simulink model "Model_RB_APF_WF_VO_withFairRules"  (R2024b)
settings: Solver=FixedStepAuto  StartTime=0.0  StopTime=150  FixedStep=UAVSampleTime  RelTol=1e-3
undefined symbols (not defined in the file): DroneMass, Gravity, Horizontal_Limits, Horizontal_Res, kD_pos, kD_vel, kI_pos, kI_vel, kP_pos, kP_vel, Lidar, MaxRange, N_filter, TopSpeed, UAV, Vertical_Limits, Vertical_Res, Waypoints
libraries: slpidlib x6, uavsimlib x4, robotcorelib x1, uavalgslib x1
(part 1 of 2)
settings Model: NumberOfSteps=100  PacingRate=10  Creator=The MathWorks, Inc.  LastModifiedBy=phill
settings SolverCC: AlgebraicLoopSolver=TrustRegion
settings DebuggingCC: ParameterPrecisionLossMsg=none  UnconnectedInputMsg=warning  UnconnectedOutputMsg=warning  UnconnectedLineMsg=warning
settings ModelReferenceCC: EnableRefExpFcnMdlSchedulingChecks=on
settings RTWCC: GPUComputeCapability=3.5  DLArmComputeVersion=19.05

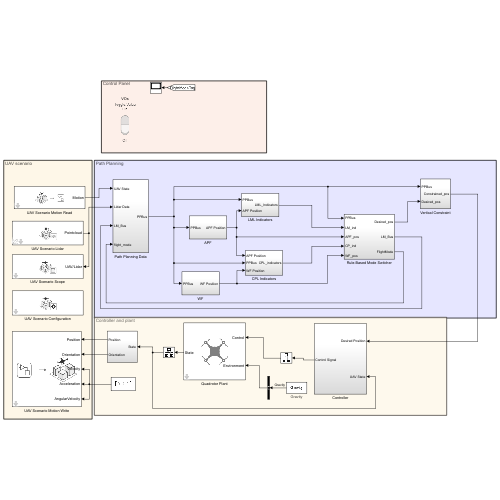
[thumbnail: Simulink's stored preview of the top-level diagram]
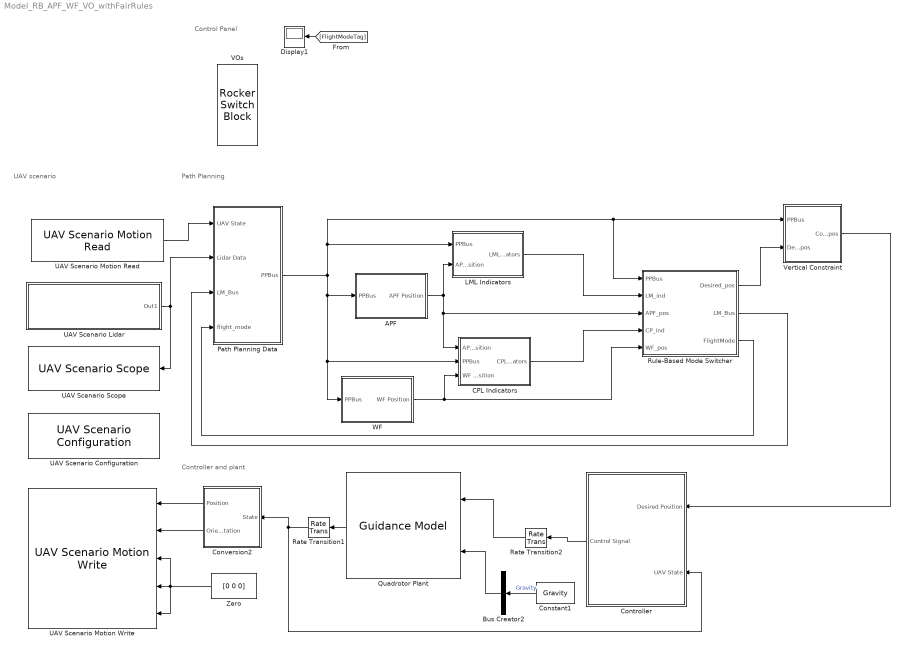
== system Model_RB_APF_WF_VO_withFairRules ==
  note: Path Planning
  note: UAV scenario
  note: Controller and plant
  note: Control Panel
  APF : Subsystem
  Bus Creator2 : BusCreator  Inputs=1  OutDataTypeStr=Bus: uavGuidanceEnvironmentBus  NonVirtualBus=on
  CPL Indicators : Subsystem
  Constant1 : Constant  Value=Gravity  OutDataTypeStr=single
      settings: AttributesFormatString=%<Value>
  Controller : Subsystem
  Conversion2 : Subsystem
  Display1 : Display
  LML Indicators : Subsystem
  Path Planning Data : Subsystem
  Quadrotor Plant : uavalgslib/Guidance Model  ModelType=MultirotorGuidance  SpecifiedDataType=single  SimulateUsing=Code generation  InitialWorldPositionMultirotor=InitialPosition'  InitialWorldVelocityMultirotor=[0; 0; 0]  InitialEulerZYXMultirotor=|  InitialBodyAngularRateRPYMultirotor=[0; 0; 0]  InitialThrustMultirotor=0  InitialNorthFixedWing=0  InitialEastFixedWing=0  InitialHeightFixedWing=0  InitialAirSpeedFixedWing=0  InitialHeadingAngleFixedWing=0  InitialFlightPathAngleFixedWing=0  InitialRollAngleFixedWing=0  InitialRollAngleRateFixedWing=0  PDRollMultirotor=[100,10]  PDPitchMultirotor=[100,10]  PYawRateMultirotor=50  PThrustMultirotor=100  MassMultirotor=0.1  PHeightFixedWing=3.9  PHeadingAngleFixedWing=3.9  PFlightPathAngleFixedWing=39  PDRollFixedWing=[3402.97, 116.67]  PAirSpeedFixedWing=1  FlightPathAngleLimitsFixedWing=[-pi/2, pi/2]  StateBusName='uavGuidanceStateBus'  ControlBusName='uavGuidanceControlBus'  EnvironmentBusName='uavGuidanceEnvironmentBus'  DataType=single
      | [ 0
      | ;0;0]
  Rate Transition1 : RateTransition  OutPortSampleTime=UAVSampleTime
  Rate Transition2 : RateTransition  OutPortSampleTime=UAVSampleTime
  Rule-Based Mode Switcher : Subsystem
  UAV Scenario Configuration : uavsimlib/UAV Scenario Configuration  Priority=-1  UAVScenarioObject=MyScenario  SampleTime=0.1  UpdateParam=true  SensorMotionBusName='SensorMotionBus'  PlatformMotionBusName='PlatformMotionBus'  ScenarioMotionBusName='ScenarioMotionBus'  ScenarioMotionSignalName='ScenarioMotions'
  UAV Scenario Lidar : Subsystem  Priority=1  AncestorBlock=uavsimlib/UAV Scenario Lidar  mask(UAV Scenario Lidar){SensorName=UAV/Lidar, MaxRange=MaxRange, RangeAccuracy=0.02, AzimuthLimits=Horizontal_Limits, AzimuthResolution=Horizontal_Res, ElevationLimits=Vertical_Limits, ElevationResolution=Vertical_Res, HasNoise=off, HasOrganizedOutput=on, SampleTime=0.1}
      mask prompts: SensorName "uav:robotsluav:uavscenariolidar:SensorName"; MaxRange "uav:robotsluav:uavscenariolidar:MaxRange"; RangeAccuracy "uav:robotsluav:uavscenariolidar:RangeAccuracy"; AzimuthLimits "uav:robotsluav:uavscenariolidar:AzimuthLimits"; AzimuthResolution "uav:robotsluav:uavscenariolidar:AzimuthResolution"; ElevationLimits "uav:robotsluav:uavscenariolidar:ElevationLimits"; ElevationResolution "uav:robotsluav:uavscenariolidar:ElevationResolution"; HasNoise "uav:robotsluav:uavscenariolidar:HasNoise"; HasOrganizedOutput "uav:robotsluav:uavscenariolidar:HasOrganizedOutput"; SampleTime "uav:robotsluav:uavscenariolidar:SampleTime"
      mask help: uav:robotsluav:uavscenariolidar:Description
      mask init:
      | % Need to set sample time to a valid value before initializing with
      | % additional set_param calls
      | set_param([gcb, '/MotionData'], 'SampleTime', '-1');
      | dataSampleTime = uav.sluav.internal.scenario.mask.ScenarioLidarSensor.initialize(gcb);
      | set_param([gcb, '/MotionData'], 'SampleTime', 'dataSampleTime');
      mask Help: eval('helpview("uav","uavScenarioLidar")');
      mask TypeOptions SensorName: LidarSensor/SensorName
      mask TypeOptions MaxRange: LidarSensor/MaxRange
      mask TypeOptions RangeAccuracy: LidarSensor/RangeAccuracy
      mask TypeOptions AzimuthLimits: LidarSensor/AzimuthLimits
      mask TypeOptions AzimuthResolution: LidarSensor/AzimuthResolution
      mask TypeOptions ElevationLimits: LidarSensor/ElevationLimits
      mask TypeOptions ElevationResolution: LidarSensor/ElevationResolution
      mask TypeOptions HasNoise: LidarSensor/HasNoise
      mask TypeOptions HasOrganizedOutput: LidarSensor/HasOrganizedOutput
      mask TypeOptions SampleTime: LidarSensor/SampleTime
      mask DialogControl SensorName Prompt: Sensor name:
      mask DialogControl SelectBtn Prompt: uav:robotsluav:uavscenarioconfig:SelectBtnPrompt
      mask DialogControl SelectBtn Callback: uav.sluav.internal.scenario.mask.ScenarioLidarSensor.selectBtnCallback(gcb);
      mask DialogControl MaxRange Prompt: Max range (m):
      mask DialogControl RangeAccuracy Prompt: Range accuracy (m):
      mask DialogControl AzimuthLimits Prompt: Azimuthal limits (deg):
      mask DialogControl AzimuthResolution Prompt: Azimuthal resolution (deg):
      mask DialogControl ElevationLimits Prompt: Elevation limits (deg):
      mask DialogControl ElevationResolution Prompt: Elevation resolution (deg):
      mask DialogControl HasNoise Prompt: Add noise to measurement.
      mask DialogControl HasOrganizedOutput Prompt: Output organized point cloud locations.
      mask DialogControl SampleTime Prompt: Sample Time:
      mask Display: port_label('output', 1, 'Pointcloud');
  UAV Scenario Motion Read : uavsimlib/UAV Scenario Motion Read  Priority=1  EntityName='UAV'  ReferenceFrame=ENU  OutputWind=off
  UAV Scenario Motion Write : uavsimlib/UAV Scenario Motion Write  Priority=0  PlatName='UAV'  ReferenceFrame=ENU
  UAV Scenario Scope : uavsimlib/UAV Scenario Scope  Priority=1  SensorNameTable={ 'UAV/Lidar', 'on' }  SampleTime=.1
  VOs : RockerSwitchBlock
      settings: Values={{'Off', 'On'}, [0 1]}
  Vertical Constraint : Subsystem
  WF : Subsystem
  Zero : Constant  Value=[0 0 0]  OutDataTypeStr=Inherit: Inherit via back propagation
  wires:
  Controller/1(Control Signal) -> Rate Transition2/1
  Rate Transition2/1 -> Quadrotor Plant/1
  Rate Transition1/1 -> Controller/2(UAV State), Conversion2/1(State)
  Quadrotor Plant/1 -> Rate Transition1/1
  Bus Creator2/1 -> Quadrotor Plant/2
  Constant1/1 -> Bus Creator2/1  "Gravity"
  UAV Scenario Motion Read/1 -> Path Planning Data/1(UAV State)
  UAV Scenario Lidar/1(Out1) -> UAV Scenario Scope/1, Path Planning Data/2(Lidar Data)
  Conversion2/1(Position) -> UAV Scenario Motion Write/1
  Conversion2/2(Orientation) -> UAV Scenario Motion Write/2
  Zero/1 -> UAV Scenario Motion Write/3, UAV Scenario Motion Write/4, UAV Scenario Motion Write/5
  APF/1(APF Position) -> Rule-Based Mode Switcher/3(APF_pos), CPL Indicators/1(APF Position), LML Indicators/2(APF Position)
  WF/1(WF Position) -> Rule-Based Mode Switcher/5(WF_pos), CPL Indicators/3(WF Position)
  Vertical Constraint/1(Constrained_pos) -> Controller/1(Desired Position)
  [FlightModeTag] -> Display1/1
  Path Planning Data/1(PPBus) -> LML Indicators/1(PPBus), Rule-Based Mode Switcher/1(PPBus), Vertical Constraint/1(PPBus), CPL Indicators/2(PPBus), WF/1(PPBus), APF/1(PPBus)
  CPL Indicators/1(CPL_indicators) -> Rule-Based Mode Switcher/4(CP_ind)
  Rule-Based Mode Switcher/1(Desired_pos) -> Vertical Constraint/2(Desired_pos)
  Rule-Based Mode Switcher/3(FlightMode) -> Path Planning Data/4(flight_mode)
  Rule-Based Mode Switcher/2(LM_Bus) -> Path Planning Data/3(LM_Bus)
  LML Indicators/1(LML_Indicators) -> Rule-Based Mode Switcher/2(LM_ind)

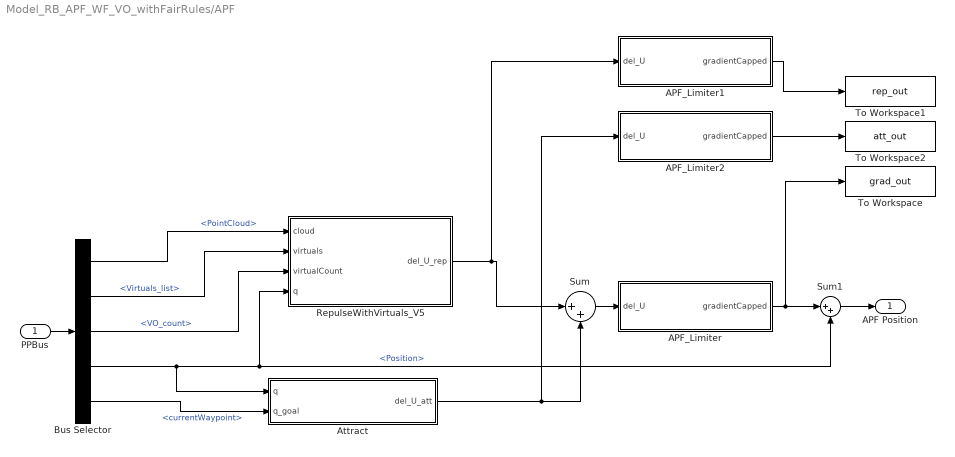
== system Model_RB_APF_WF_VO_withFairRules/APF ==
  PPBus : Inport
  APF_Limiter : MATLAB Function  TreatAsAtomicUnit=on
  APF_Limiter1 : MATLAB Function  TreatAsAtomicUnit=on
  APF_Limiter2 : MATLAB Function  TreatAsAtomicUnit=on
  Attract : MATLAB Function  TreatAsAtomicUnit=on
  Bus Selector : BusSelector  OutputSignals=PointCloud,VO_Bus.Virtuals_list,VO_Bus.VO_count,Position,currentWaypoint
  RepulseWithVirtuals_V5 : MATLAB Function  TreatAsAtomicUnit=on
  Sum : Sum  Inputs=|++
  Sum1 : Sum  Inputs=|++
  To Workspace : ToWorkspace  VariableName=grad_out  SampleTime=-1
      settings: Decimation=Plot_decimation_1s
  To Workspace1 : ToWorkspace  VariableName=rep_out  SampleTime=-1
      settings: Decimation=Plot_decimation_1s
  To Workspace2 : ToWorkspace  VariableName=att_out  SampleTime=-1
      settings: Decimation=Plot_decimation_1s
  APF Position : Outport
  wires:
  PPBus/1 -> Bus Selector/1
  Sum1/1 -> APF Position/1
  Sum/1 -> APF_Limiter/1(del_U)
  APF_Limiter/1(gradientCapped) -> Sum1/1, To Workspace/1
  Attract/1(del_U_att) -> APF_Limiter2/1(del_U), Sum/2
  RepulseWithVirtuals_V5/1(del_U_rep) -> APF_Limiter1/1(del_U), Sum/1
  Bus Selector/1 -> RepulseWithVirtuals_V5/1(cloud)  "<PointCloud>"
  Bus Selector/4 -> RepulseWithVirtuals_V5/4(q), Sum1/2, Attract/1(q)  "<Position>"
  Bus Selector/5 -> Attract/2(q_goal)  "<currentWaypoint>"
  APF_Limiter1/1(gradientCapped) -> To Workspace1/1
  APF_Limiter2/1(gradientCapped) -> To Workspace2/1
  Bus Selector/2 -> RepulseWithVirtuals_V5/2(virtuals)  "<Virtuals_list>"
  Bus Selector/3 -> RepulseWithVirtuals_V5/3(virtualCount)  "<VO_count>"

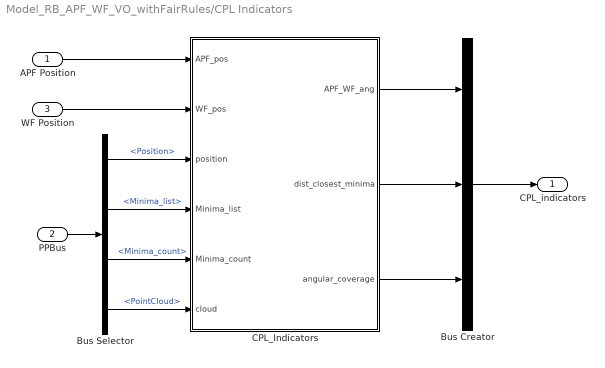
== system Model_RB_APF_WF_VO_withFairRules/CPL Indicators ==
  APF Position : Inport
  PPBus : Inport  Port=2
  WF Position : Inport  Port=3
  Bus Creator : BusCreator  Inputs=3
  Bus Selector : BusSelector  OutputSignals=Position,LM_Bus.Minima_list,LM_Bus.Minima_count,PointCloud
  CPL_Indicators : MATLAB Function  TreatAsAtomicUnit=on
  CPL_indicators : Outport
  wires:
  PPBus/1 -> Bus Selector/1
  Bus Selector/1 -> CPL_Indicators/3(position)  "<Position>"
  Bus Selector/3 -> CPL_Indicators/5(Minima_count)  "<Minima_count>"
  Bus Selector/2 -> CPL_Indicators/4(Minima_list)  "<Minima_list>"
  Bus Selector/4 -> CPL_Indicators/6(cloud)  "<PointCloud>"
  Bus Creator/1 -> CPL_indicators/1
  CPL_Indicators/2(dist_closest_minima) -> Bus Creator/2
  CPL_Indicators/3(angular_coverage) -> Bus Creator/3
  WF Position/1 -> CPL_Indicators/2(WF_pos)
  APF Position/1 -> CPL_Indicators/1(APF_pos)
  CPL_Indicators/1(APF_WF_ang) -> Bus Creator/1

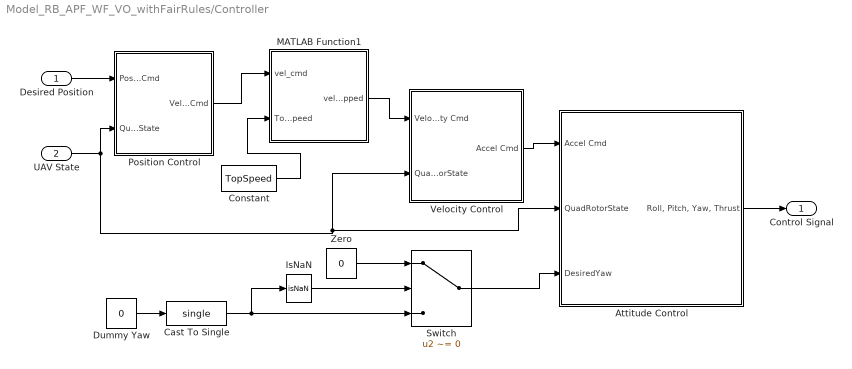
== system Model_RB_APF_WF_VO_withFairRules/Controller ==
  Desired Position : Inport
  UAV State : Inport  Port=2
  Attitude Control : Subsystem
  Cast To Single : DataTypeConversion  OutDataTypeStr=single  SaturateOnIntegerOverflow=off  RndMeth=Floor
  Constant : Constant  Value=TopSpeed
  Dummy Yaw : Constant  Value=0
  IsNaN : RelationalOperator  Operator=isNaN  OutDataTypeStr=boolean  RndMeth=Simplest  InputSameDT=off
  MATLAB Function1 : MATLAB Function  TreatAsAtomicUnit=on
  Position Control : Subsystem
  Switch : Switch  Criteria=u2 ~= 0  SaturateOnIntegerOverflow=off  InputSameDT=off
  Velocity Control : Subsystem
  Zero : Constant  Value=0  OutDataTypeStr=Inherit: Inherit via back propagation
  Control Signal : Outport
  wires:
  Desired Position/1 -> Position Control/1(PositionCmd)
  Velocity Control/1(Accel Cmd) -> Attitude Control/1(Accel Cmd)
  Attitude Control/1("Roll, Pitch, Yaw, Thrust") -> Control Signal/1
  UAV State/1 -> Position Control/2(QuadRotorState), Velocity Control/2(QuadRotorState), Attitude Control/2(QuadRotorState)
  Zero/1 -> Switch/1
  IsNaN/1 -> Switch/2
  Cast To Single/1 -> IsNaN/1, Switch/3
  Switch/1 -> Attitude Control/3(DesiredYaw)
  Dummy Yaw/1 -> Cast To Single/1
  Position Control/1(Velocity Cmd) -> MATLAB Function1/1(vel_cmd)
  MATLAB Function1/1(vel_capped) -> Velocity Control/1(Velocity Cmd)
  Constant/1 -> MATLAB Function1/2(TopSpeed)

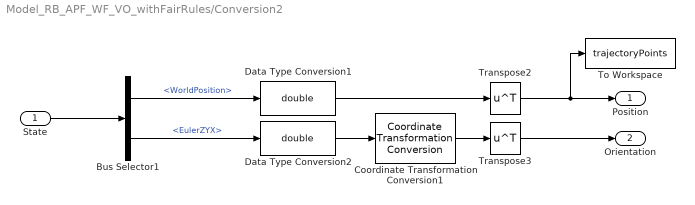
== system Model_RB_APF_WF_VO_withFairRules/Conversion2 ==
  State : Inport
  Bus Selector1 : BusSelector  OutputSignals=WorldPosition,EulerZYX
  Coordinate Transformation Conversion1 : robotcorelib/Coordinate Transformation Conversion  InputRepresentation=Euler Angles  InputEulerSequence=ZYX  ShowTrVecInputPort=on  OutputRepresentation=Quaternion  OutputEulerSequence=ZYX  ShowTrVecOutputPort=on  SimulateUsing=Code generation
  Data Type Conversion1 : DataTypeConversion  OutDataTypeStr=double  SaturateOnIntegerOverflow=off  RndMeth=Floor
  Data Type Conversion2 : DataTypeConversion  OutDataTypeStr=double  SaturateOnIntegerOverflow=off  RndMeth=Floor
  To Workspace : ToWorkspace  VariableName=trajectoryPoints  SampleTime=-1
  Transpose2 : Math  Operator=transpose
  Transpose3 : Math  Operator=transpose
  Position : Outport
  Orientation : Outport  Port=2
  wires:
  State/1 -> Bus Selector1/1
  Transpose2/1 -> To Workspace/1, Position/1
  Bus Selector1/1 -> Data Type Conversion1/1  "<WorldPosition>"
  Data Type Conversion2/1 -> Coordinate Transformation Conversion1/1
  Bus Selector1/2 -> Data Type Conversion2/1  "<EulerZYX>"
  Coordinate Transformation Conversion1/1 -> Transpose3/1
  Transpose3/1 -> Orientation/1
  Data Type Conversion1/1 -> Transpose2/1

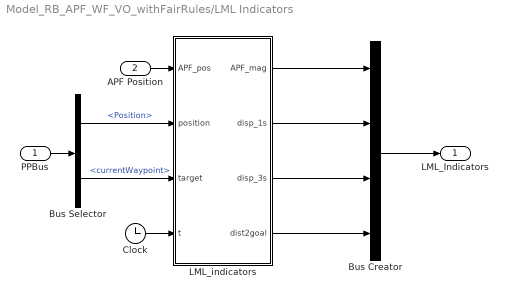
== system Model_RB_APF_WF_VO_withFairRules/LML Indicators ==
  PPBus : Inport
  APF Position : Inport  Port=2
  Bus Creator : BusCreator  Inputs=4
  Bus Selector : BusSelector  OutputSignals=Position,currentWaypoint
  Clock : Clock
  LML_indicators : MATLAB Function  TreatAsAtomicUnit=on
  LML_Indicators : Outport
  wires:
  PPBus/1 -> Bus Selector/1
  Bus Selector/1 -> LML_indicators/2(position)  "<Position>"
  Clock/1 -> LML_indicators/4(t)
  LML_indicators/3(disp_3s) -> Bus Creator/3
  LML_indicators/2(disp_1s) -> Bus Creator/2
  APF Position/1 -> LML_indicators/1(APF_pos)
  LML_indicators/1(APF_mag) -> Bus Creator/1
  Bus Creator/1 -> LML_Indicators/1
  Bus Selector/2 -> LML_indicators/3(target)  "<currentWaypoint>"
  LML_indicators/4(dist2goal) -> Bus Creator/4

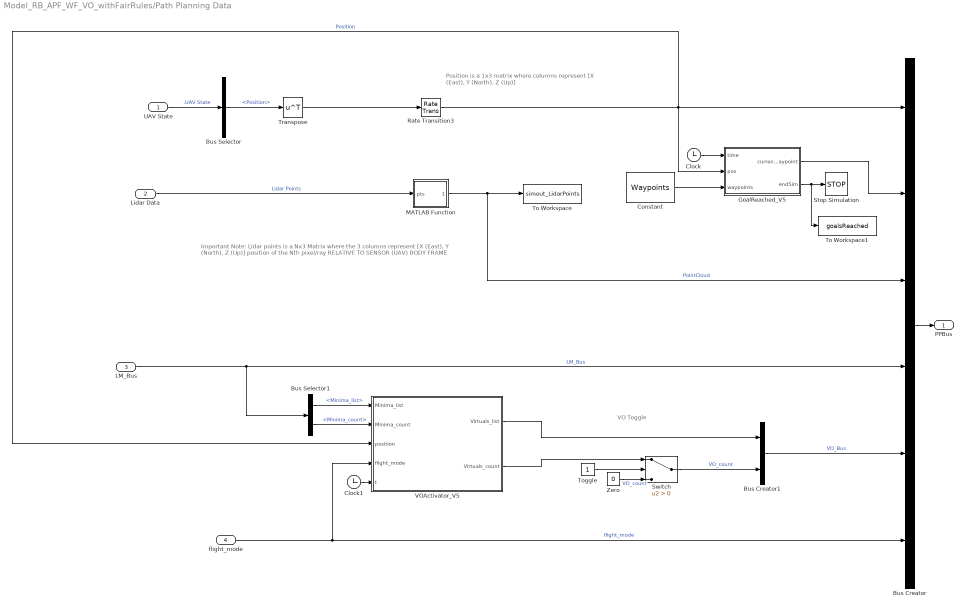
== system Model_RB_APF_WF_VO_withFairRules/Path Planning Data ==
  note: VO Toggle
  note: Position is a 1x3 matrix where columns represent [X (East), Y (North), Z (Up)]
  note: Important Note:
      | Lidar points is a Nx3 Matrix where the 3 columns represent [X (East), Y (North), Z (Up)] position of the Nth pixel/ray RELATIVE TO SENSOR (UAV) BODY FRAME
  UAV State : Inport
  Lidar Data : Inport  Port=2
  LM_Bus : Inport  Port=3
  flight_mode : Inport  Port=4
  Bus Creator : BusCreator  Inputs=6
  Bus Creator1 : BusCreator  Inputs=2
  Bus Selector : BusSelector  OutputSignals=Position
  Bus Selector1 : BusSelector  OutputSignals=Minima_list,Minima_count
  Clock : Clock
  Clock1 : Clock
  Constant : Constant  Value=Waypoints  VectorParams1D=off
  GoalReached_V5 : MATLAB Function  TreatAsAtomicUnit=on
  MATLAB Function : MATLAB Function  TreatAsAtomicUnit=on
  Rate Transition3 : RateTransition  OutPortSampleTime=.1
  Stop Simulation : Stop
  Switch : Switch  Criteria=u2 > Threshold  SaturateOnIntegerOverflow=off  InputSameDT=off
  To Workspace : ToWorkspace  VariableName=simout_LidarPoints  SampleTime=-1
  To Workspace1 : ToWorkspace  VariableName=goalsReached  SaveFormat=Timeseries  SampleTime=-1
  Toggle : Constant
  Transpose : Math  Operator=transpose
  VOActivator_V5 : MATLAB Function  TreatAsAtomicUnit=on
  Zero : Constant  Value=0
  PPBus : Outport
  wires:
  Bus Selector/1 -> Transpose/1  "<Position>"
  UAV State/1 -> Bus Selector/1  ".UAV State"
  Lidar Data/1 -> MATLAB Function/1(pts)  "Lidar Points"
  MATLAB Function/1(points) -> Bus Creator/3, To Workspace/1  "PointCloud"
  Rate Transition3/1 -> GoalReached_V5/2(pos), VOActivator_V5/3(position), Bus Creator/1  "Position"
  Transpose/1 -> Rate Transition3/1
  Bus Creator/1 -> PPBus/1
  Constant/1 -> GoalReached_V5/3(waypoints)
  Clock/1 -> GoalReached_V5/1(time)
  Toggle/1 -> Switch/2
  Switch/1 -> Bus Creator1/2  "VO_count"
  Zero/1 -> Switch/3  "VO_count"
  Bus Creator1/1 -> Bus Creator/5  "VO_Bus"
  LM_Bus/1 -> Bus Selector1/1, Bus Creator/4  "LM_Bus"
  VOActivator_V5/1(Virtuals_list) -> Bus Creator1/1
  VOActivator_V5/2(Virtuals_count) -> Switch/1
  flight_mode/1 -> VOActivator_V5/4(flight_mode), Bus Creator/6  "flight_mode"
  Bus Selector1/1 -> VOActivator_V5/1(Minima_list)  "<Minima_list>"
  Bus Selector1/2 -> VOActivator_V5/2(Minima_count)  "<Minima_count>"
  Clock1/1 -> VOActivator_V5/5(t)
  GoalReached_V5/1(currentWaypoint) -> Bus Creator/2
  GoalReached_V5/2(endSim) -> To Workspace1/1, Stop Simulation/1

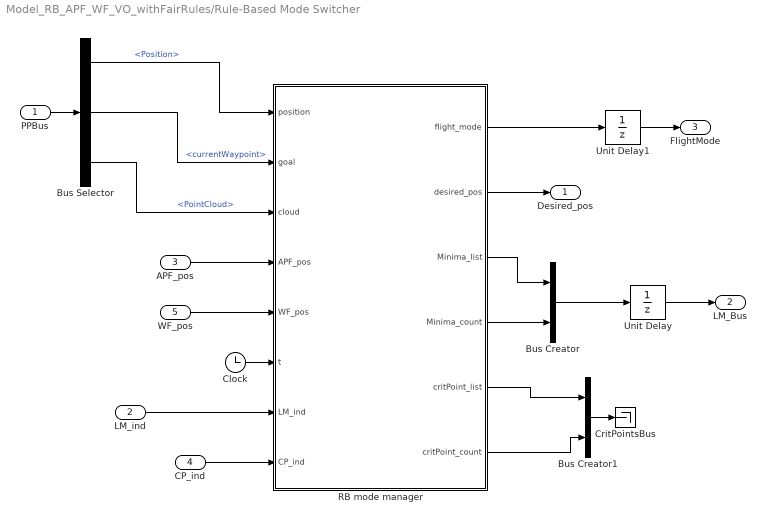
== system Model_RB_APF_WF_VO_withFairRules/Rule-Based Mode Switcher ==
  PPBus : Inport
  LM_ind : Inport  Port=2
  APF_pos : Inport  Port=3
  CP_ind : Inport  Port=4
  WF_pos : Inport  Port=5
  Bus Creator : BusCreator  Inputs=2
  Bus Creator1 : BusCreator  Inputs=2
  Bus Selector : BusSelector  OutputSignals=Position,currentWaypoint,PointCloud
  Clock : Clock
  CritPointsBus : Terminator
  RB mode manager : MATLAB Function  TreatAsAtomicUnit=on
  Unit Delay : UnitDelay  InitialCondition=1  SampleTime=-1  HasFrameUpgradeWarning=on
  Unit Delay1 : UnitDelay  InitialCondition=1  SampleTime=-1  HasFrameUpgradeWarning=on
  Desired_pos : Outport
  LM_Bus : Outport  Port=2
  FlightMode : Outport  Port=3
  wires:
  APF_pos/1 -> RB mode manager/4(APF_pos)
  WF_pos/1 -> RB mode manager/5(WF_pos)
  PPBus/1 -> Bus Selector/1
  Bus Selector/1 -> RB mode manager/1(position)  "<Position>"
  Bus Selector/2 -> RB mode manager/2(goal)  "<currentWaypoint>"
  Bus Selector/3 -> RB mode manager/3(cloud)  "<PointCloud>"
  RB mode manager/2(desired_pos) -> Desired_pos/1
  RB mode manager/3(Minima_list) -> Bus Creator/1
  RB mode manager/4(Minima_count) -> Bus Creator/2
  RB mode manager/5(critPoint_list) -> Bus Creator1/1
  RB mode manager/6(critPoint_count) -> Bus Creator1/2
  Clock/1 -> RB mode manager/6(t)
  Bus Creator1/1 -> CritPointsBus/1
  Bus Creator/1 -> Unit Delay/1
  Unit Delay/1 -> LM_Bus/1
  RB mode manager/1(flight_mode) -> Unit Delay1/1
  Unit Delay1/1 -> FlightMode/1
  LM_ind/1 -> RB mode manager/7(LM_ind)
  CP_ind/1 -> RB mode manager/8(CP_ind)

== system Model_RB_APF_WF_VO_withFairRules/UAV Scenario Lidar ==
  LidarSensor : MATLABSystem  System=uav.sluav.internal.system.UAVScenarioLidarGenerator  SensorName=UAV/Lidar  MaxRange=MaxRange  RangeAccuracy=RangeAccuracy  AzimuthResolution=AzimuthResolution  ElevationResolution=ElevationResolution  AzimuthLimits=AzimuthLimits  ElevationLimits=ElevationLimits  HasNoise=off  HasOrganizedOutput=on  SampleTime=SampleTime
      mask Type: uav.sluav.internal.system.UAVScenarioLidarGenerator
      mask Display:
      | disp('UAVScenarioLidarGenerator');
      | port_label('input',1,'motions');
      | port_label('output',1,'y');
  MotionData : DataStoreRead  DataStoreName=ScenarioMotions  SampleTime=dataSampleTime  IndexOptions=Index vector (dialog)  Indices=1  OutputSizes=1
  Out1 : Outport
  wires:
  LidarSensor/1 -> Out1/1
  MotionData/1 -> LidarSensor/1

== system Model_RB_APF_WF_VO_withFairRules/Vertical Constraint ==
  PPBus : Inport
  Desired_pos : Inport  Port=2
  Bus Selector : BusSelector  OutputSignals=currentWaypoint
  MATLAB Function : MATLAB Function  TreatAsAtomicUnit=on
  Constrained_pos : Outport
  wires:
  Desired_pos/1 -> MATLAB Function/1(desired_pos)
  MATLAB Function/1(constrained_pos) -> Constrained_pos/1
  PPBus/1 -> Bus Selector/1
  Bus Selector/1 -> MATLAB Function/2(current_waypoint)  "<currentWaypoint>"

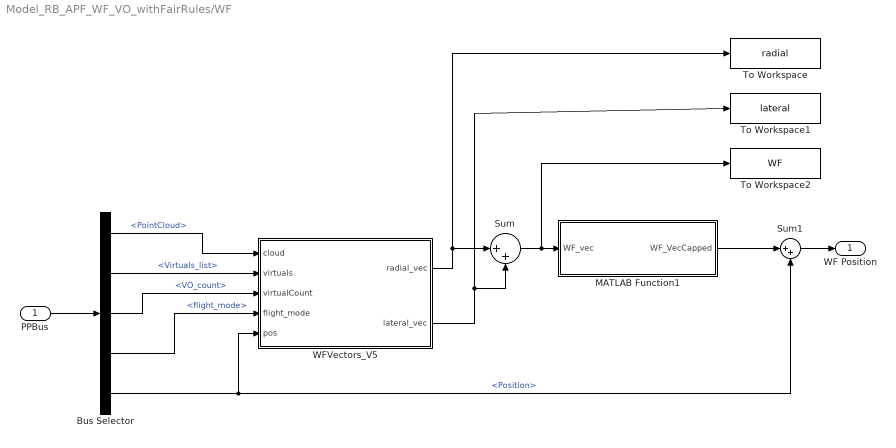
== system Model_RB_APF_WF_VO_withFairRules/WF ==
  PPBus : Inport
  Bus Selector : BusSelector  OutputSignals=PointCloud,VO_Bus.Virtuals_list,VO_Bus.VO_count,flight_mode,Position
  MATLAB Function1 : MATLAB Function  TreatAsAtomicUnit=on
  Sum : Sum  Inputs=|++
  Sum1 : Sum  Inputs=|++
  To Workspace : ToWorkspace  VariableName=radial  SampleTime=-1
      settings: Decimation=Plot_decimation_1s
  To Workspace1 : ToWorkspace  VariableName=lateral  SampleTime=-1
      settings: Decimation=Plot_decimation_1s
  To Workspace2 : ToWorkspace  VariableName=WF  SampleTime=-1
      settings: Decimation=Plot_decimation_1s
  WFVectors_V5 : MATLAB Function  TreatAsAtomicUnit=on
  WF Position : Outport
  wires:
  Sum1/1 -> WF Position/1
  PPBus/1 -> Bus Selector/1
  Sum/1 -> To Workspace2/1, MATLAB Function1/1(WF_vec)
  WFVectors_V5/2(lateral_vec) -> To Workspace1/1, Sum/2
  Bus Selector/4 -> WFVectors_V5/4(flight_mode)  "<flight_mode>"
  Bus Selector/1 -> WFVectors_V5/1(cloud)  "<PointCloud>"
  MATLAB Function1/1(WF_VecCapped) -> Sum1/1
  Bus Selector/5 -> WFVectors_V5/5(pos), Sum1/2  "<Position>"
  WFVectors_V5/1(radial_vec) -> To Workspace/1, Sum/1
  Bus Selector/2 -> WFVectors_V5/2(virtuals)  "<Virtuals_list>"
  Bus Selector/3 -> WFVectors_V5/3(virtualCount)  "<VO_count>"

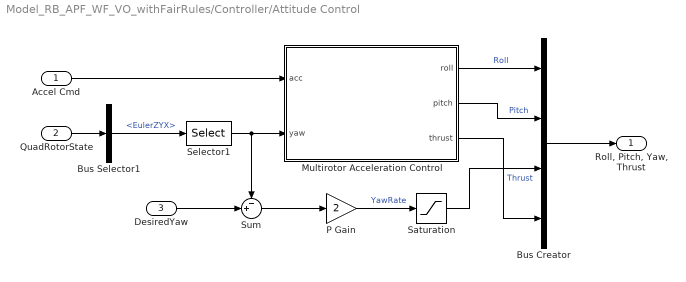
== system Model_RB_APF_WF_VO_withFairRules/Controller/Attitude Control ==
  Accel Cmd : Inport
  QuadRotorState : Inport  Port=2
  DesiredYaw : Inport  Port=3
  Bus Creator : BusCreator  Inputs=4  OutDataTypeStr=Bus: uavGuidanceControlBus  NonVirtualBus=on
      settings: InheritFromInputs=off
  Bus Selector1 : BusSelector  OutputSignals=EulerZYX
  Multirotor Acceleration Control : MATLAB Function  TreatAsAtomicUnit=on
  P Gain : Gain  Gain=2
  Saturation : Saturate
  Selector1 : Selector  InputPortWidth=3  IndexOptions=Index vector (dialog)  Indices=[1]  OutputSizes=1
  Sum : Sum  Inputs=-+|
  "Roll, Pitch, Yaw, Thrust" : Outport
  wires:
  Selector1/1 -> Multirotor Acceleration Control/2(yaw), Sum/1
  Bus Creator/1 -> "Roll, Pitch, Yaw, Thrust"/1
  Sum/1 -> P Gain/1
  Multirotor Acceleration Control/1(roll) -> Bus Creator/1  "Roll"
  Multirotor Acceleration Control/2(pitch) -> Bus Creator/2  "Pitch"
  Multirotor Acceleration Control/3(thrust) -> Bus Creator/4  "Thrust"
  P Gain/1 -> Saturation/1  "YawRate"
  Accel Cmd/1 -> Multirotor Acceleration Control/1(acc)
  QuadRotorState/1 -> Bus Selector1/1
  Bus Selector1/1 -> Selector1/1  "<EulerZYX>"
  Saturation/1 -> Bus Creator/3
  DesiredYaw/1 -> Sum/2

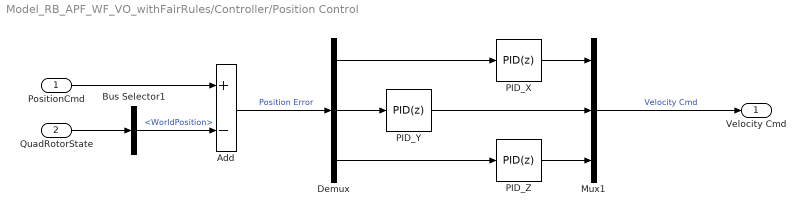
== system Model_RB_APF_WF_VO_withFairRules/Controller/Position Control ==
  PositionCmd : Inport
  QuadRotorState : Inport  Port=2
  Add : Sum  Inputs=+-
  Bus Selector1 : BusSelector  OutputSignals=WorldPosition
  Demux : Demux  Outputs=3
  Mux1 : Mux  Inputs=3
  PID_X : slpidlib/PID Controller  Controller=PID  Form=Parallel  TimeDomain=Discrete-time  UseExternalTs=off  SampleTime=-1  IntegratorMethod=Forward Euler  FilterMethod=Forward Euler  ControllerParametersSource=internal  P=kP_pos  I=kI_pos  UseKiTs=off  D=kD_pos  UseExternalDerivativeSource=off  N=N_filter  UseFilter=on  TunerSelectOption=Transfer Function Based (PID Tuner App)  InitialConditionSource=internal  InitialConditionForIntegrator=0  InitialConditionForFilter=0  DifferentiatorICPrevScaledInput=0  ExternalReset=none  TrackingMode=off  Kt=1  LimitOutput=on  SatLimitsSource=internal  UpperSaturationLimit=3  LowerSaturationLimit=-3  LinearizeAsGain=on  AntiWindupMode=clamping  Kb=1  LimitIntegrator=off  UpperIntegratorSaturationLimit=inf  LowerIntegratorSaturationLimit=-inf  POutMin=[]  POutMax=[]  IOutMin=[]  IOutMax=[]  DOutMin=[]  DOutMax=[]  NOutMin=[]  NOutMax=[]  SumOutMin=[]  SumOutMax=[]  SaturationOutMin=[]  SaturationOutMax=[]  PParamMin=[]  PParamMax=[]  IParamMin=[]  IParamMax=[]  DParamMin=[]  DParamMax=[]  NParamMin=[]  NParamMax=[]  KbParamMin=[]  KbParamMax=[]  KtParamMin=[]  KtParamMax=[]  KbOutMin=[]  KbOutMax=[]  KtOutMin=[]  KtOutMax=[]  IntegratorOutMin=[]  IntegratorOutMax=[]  FilterOutMin=[]  FilterOutMax=[]  SumI1OutMin=SumI1OutMin  SumI1OutMax=SumI1OutMax  SumI2OutMin=[]  SumI2OutMax=[]  SumI3OutMin=[]  SumI3OutMax=[]  SumI4OutMin=[]  SumI4OutMax=[]  SumDOutMin=[]  SumDOutMax=[]  DifferentiatorOutMin=[]  DifferentiatorOutMax=[]  FilterDiffOutCoefMin=[]  FilterDiffOutCoefMax=[]  ReciprocalOutMin=[]  ReciprocalOutMax=[]  SumDenOutMin=[]  SumDenOutMax=[]  SumNumOutMin=[]  SumNumOutMax=[]  DivideOutMin=[]  DivideOutMax=[]  UdiffTsProdOutMin=[]  UdiffTsProdOutMax=[]  NTsProdOutMin=[]  NTsProdOutMax=[]  UintegralTsProdOutMin=[]  UintegralTsProdOutMax=[]  UngainTsProdOutMin=[]  UngainTsProdOutMax=[]  ClampingZeroOutDataTypeStr=Inherit: Inherit via back propagation  ClampingZeroOutMin=[]  ClampingZeroOutMax=[]  FilterDenConstantOutDataTypeStr=Inherit: Inherit via back propagation  FilterDenConstantOutMin=[]  FilterDenConstantOutMax=[]  PCopyOutDataTypeStr=Inherit: Inherit via back propagation  PCopyOutMin=[]  PCopyOutMax=[]  NCopyOutDataTypeStr=Inherit: Inherit via back propagation  NCopyOutMin=[]  NCopyOutMax=[]  IntegratorContinuousStateAttributes=''  IntegratorStateMustResolveToSignalObject=off  IntegratorRTWStateStorageClass=Auto  FilterContinuousStateAttributes=''  FilterStateMustResolveToSignalObject=off  FilterRTWStateStorageClass=Auto  ParallelPVariant=InternalParameters  IdealPVariant=Disabled  IVariant=InternalParameters  DVariant=InternalParameters  IntegratorVariant=Discrete  SatVariant=Enabled  AWVariant=DiscClampingParallel  PCopyVariant=Disabled  TRVariant=Disabled  FdbkBlocksVariant=Forward  IdealPFdbkVariant=Disabled  SatFdbkVariant=Disabled  DerivativeFilterVariant=ForwardEulerFilter  NVariant=InternalParameters  NCopyVariant=Disabled  FilterICVariant=InternalICsFilter  IntegratorICVariant=InternalICs  ExternalResetVariant=Disabled  TRSumVariant=Passthrough  SumFdbkVariant=Disabled  SumVariant=Sum_PID  TsampFilterVariant=InternalTs  TsampNgainVariant=Passthrough  TsampIntegralVariant=Disabled_SignalSpec  ExternalSaturationOutDataTypeStr=Inherit: Same as second input  DerivativeSourceVariant=ErrorSignal  PreIntVariant=InternalPreInt
      settings: AttributesFormatString=P: %<P>, I: %<I>, D:%<D>
  PID_Y : slpidlib/PID Controller  Controller=PID  Form=Parallel  TimeDomain=Discrete-time  UseExternalTs=off  SampleTime=-1  IntegratorMethod=Forward Euler  FilterMethod=Forward Euler  ControllerParametersSource=internal  P=kP_pos  I=kI_pos  UseKiTs=off  D=kD_pos  UseExternalDerivativeSource=off  N=N_filter  UseFilter=on  TunerSelectOption=Transfer Function Based (PID Tuner App)  InitialConditionSource=internal  InitialConditionForIntegrator=0  InitialConditionForFilter=0  DifferentiatorICPrevScaledInput=0  ExternalReset=none  TrackingMode=off  Kt=1  LimitOutput=on  SatLimitsSource=internal  UpperSaturationLimit=3  LowerSaturationLimit=-3  LinearizeAsGain=on  AntiWindupMode=clamping  Kb=1  LimitIntegrator=off  UpperIntegratorSaturationLimit=inf  LowerIntegratorSaturationLimit=-inf  POutMin=[]  POutMax=[]  IOutMin=[]  IOutMax=[]  DOutMin=[]  DOutMax=[]  NOutMin=[]  NOutMax=[]  SumOutMin=[]  SumOutMax=[]  SaturationOutMin=[]  SaturationOutMax=[]  PParamMin=[]  PParamMax=[]  IParamMin=[]  IParamMax=[]  DParamMin=[]  DParamMax=[]  NParamMin=[]  NParamMax=[]  KbParamMin=[]  KbParamMax=[]  KtParamMin=[]  KtParamMax=[]  KbOutMin=[]  KbOutMax=[]  KtOutMin=[]  KtOutMax=[]  IntegratorOutMin=[]  IntegratorOutMax=[]  FilterOutMin=[]  FilterOutMax=[]  SumI1OutMin=SumI1OutMin  SumI1OutMax=SumI1OutMax  SumI2OutMin=[]  SumI2OutMax=[]  SumI3OutMin=[]  SumI3OutMax=[]  SumI4OutMin=[]  SumI4OutMax=[]  SumDOutMin=[]  SumDOutMax=[]  DifferentiatorOutMin=[]  DifferentiatorOutMax=[]  FilterDiffOutCoefMin=[]  FilterDiffOutCoefMax=[]  ReciprocalOutMin=[]  ReciprocalOutMax=[]  SumDenOutMin=[]  SumDenOutMax=[]  SumNumOutMin=[]  SumNumOutMax=[]  DivideOutMin=[]  DivideOutMax=[]  UdiffTsProdOutMin=[]  UdiffTsProdOutMax=[]  NTsProdOutMin=[]  NTsProdOutMax=[]  UintegralTsProdOutMin=[]  UintegralTsProdOutMax=[]  UngainTsProdOutMin=[]  UngainTsProdOutMax=[]  ClampingZeroOutDataTypeStr=Inherit: Inherit via back propagation  ClampingZeroOutMin=[]  ClampingZeroOutMax=[]  FilterDenConstantOutDataTypeStr=Inherit: Inherit via back propagation  FilterDenConstantOutMin=[]  FilterDenConstantOutMax=[]  PCopyOutDataTypeStr=Inherit: Inherit via back propagation  PCopyOutMin=[]  PCopyOutMax=[]  NCopyOutDataTypeStr=Inherit: Inherit via back propagation  NCopyOutMin=[]  NCopyOutMax=[]  IntegratorContinuousStateAttributes=''  IntegratorStateMustResolveToSignalObject=off  IntegratorRTWStateStorageClass=Auto  FilterContinuousStateAttributes=''  FilterStateMustResolveToSignalObject=off  FilterRTWStateStorageClass=Auto  ParallelPVariant=InternalParameters  IdealPVariant=Disabled  IVariant=InternalParameters  DVariant=InternalParameters  IntegratorVariant=Discrete  SatVariant=Enabled  AWVariant=DiscClampingParallel  PCopyVariant=Disabled  TRVariant=Disabled  FdbkBlocksVariant=Forward  IdealPFdbkVariant=Disabled  SatFdbkVariant=Disabled  DerivativeFilterVariant=ForwardEulerFilter  NVariant=InternalParameters  NCopyVariant=Disabled  FilterICVariant=InternalICsFilter  IntegratorICVariant=InternalICs  ExternalResetVariant=Disabled  TRSumVariant=Passthrough  SumFdbkVariant=Disabled  SumVariant=Sum_PID  TsampFilterVariant=InternalTs  TsampNgainVariant=Passthrough  TsampIntegralVariant=Disabled_SignalSpec  ExternalSaturationOutDataTypeStr=Inherit: Same as second input  DerivativeSourceVariant=ErrorSignal  PreIntVariant=InternalPreInt
      settings: AttributesFormatString=P: %<P>, I: %<I>, D:%<D>
  PID_Z : slpidlib/PID Controller  Controller=PID  Form=Parallel  TimeDomain=Discrete-time  UseExternalTs=off  SampleTime=-1  IntegratorMethod=Forward Euler  FilterMethod=Forward Euler  ControllerParametersSource=internal  P=kP_pos  I=kI_pos  UseKiTs=off  D=kD_pos  UseExternalDerivativeSource=off  N=N_filter  UseFilter=on  TunerSelectOption=Transfer Function Based (PID Tuner App)  InitialConditionSource=internal  InitialConditionForIntegrator=0  InitialConditionForFilter=0  DifferentiatorICPrevScaledInput=0  ExternalReset=none  TrackingMode=off  Kt=1  LimitOutput=on  SatLimitsSource=internal  UpperSaturationLimit=3  LowerSaturationLimit=-3  LinearizeAsGain=on  AntiWindupMode=clamping  Kb=1  LimitIntegrator=off  UpperIntegratorSaturationLimit=inf  LowerIntegratorSaturationLimit=-inf  POutMin=[]  POutMax=[]  IOutMin=[]  IOutMax=[]  DOutMin=[]  DOutMax=[]  NOutMin=[]  NOutMax=[]  SumOutMin=[]  SumOutMax=[]  SaturationOutMin=[]  SaturationOutMax=[]  PParamMin=[]  PParamMax=[]  IParamMin=[]  IParamMax=[]  DParamMin=[]  DParamMax=[]  NParamMin=[]  NParamMax=[]  KbParamMin=[]  KbParamMax=[]  KtParamMin=[]  KtParamMax=[]  KbOutMin=[]  KbOutMax=[]  KtOutMin=[]  KtOutMax=[]  IntegratorOutMin=[]  IntegratorOutMax=[]  FilterOutMin=[]  FilterOutMax=[]  SumI1OutMin=SumI1OutMin  SumI1OutMax=SumI1OutMax  SumI2OutMin=[]  SumI2OutMax=[]  SumI3OutMin=[]  SumI3OutMax=[]  SumI4OutMin=[]  SumI4OutMax=[]  SumDOutMin=[]  SumDOutMax=[]  DifferentiatorOutMin=[]  DifferentiatorOutMax=[]  FilterDiffOutCoefMin=[]  FilterDiffOutCoefMax=[]  ReciprocalOutMin=[]  ReciprocalOutMax=[]  SumDenOutMin=[]  SumDenOutMax=[]  SumNumOutMin=[]  SumNumOutMax=[]  DivideOutMin=[]  DivideOutMax=[]  UdiffTsProdOutMin=[]  UdiffTsProdOutMax=[]  NTsProdOutMin=[]  NTsProdOutMax=[]  UintegralTsProdOutMin=[]  UintegralTsProdOutMax=[]  UngainTsProdOutMin=[]  UngainTsProdOutMax=[]  ClampingZeroOutDataTypeStr=Inherit: Inherit via back propagation  ClampingZeroOutMin=[]  ClampingZeroOutMax=[]  FilterDenConstantOutDataTypeStr=Inherit: Inherit via back propagation  FilterDenConstantOutMin=[]  FilterDenConstantOutMax=[]  PCopyOutDataTypeStr=Inherit: Inherit via back propagation  PCopyOutMin=[]  PCopyOutMax=[]  NCopyOutDataTypeStr=Inherit: Inherit via back propagation  NCopyOutMin=[]  NCopyOutMax=[]  IntegratorContinuousStateAttributes=''  IntegratorStateMustResolveToSignalObject=off  IntegratorRTWStateStorageClass=Auto  FilterContinuousStateAttributes=''  FilterStateMustResolveToSignalObject=off  FilterRTWStateStorageClass=Auto  ParallelPVariant=InternalParameters  IdealPVariant=Disabled  IVariant=InternalParameters  DVariant=InternalParameters  IntegratorVariant=Discrete  SatVariant=Enabled  AWVariant=DiscClampingParallel  PCopyVariant=Disabled  TRVariant=Disabled  FdbkBlocksVariant=Forward  IdealPFdbkVariant=Disabled  SatFdbkVariant=Disabled  DerivativeFilterVariant=ForwardEulerFilter  NVariant=InternalParameters  NCopyVariant=Disabled  FilterICVariant=InternalICsFilter  IntegratorICVariant=InternalICs  ExternalResetVariant=Disabled  TRSumVariant=Passthrough  SumFdbkVariant=Disabled  SumVariant=Sum_PID  TsampFilterVariant=InternalTs  TsampNgainVariant=Passthrough  TsampIntegralVariant=Disabled_SignalSpec  ExternalSaturationOutDataTypeStr=Inherit: Same as second input  DerivativeSourceVariant=ErrorSignal  PreIntVariant=InternalPreInt
      settings: AttributesFormatString=P: %<P>, I: %<I>, D:%<D>
  Velocity Cmd : Outport
  wires:
  Demux/3 -> PID_Z/1
  Demux/1 -> PID_X/1
  PID_Z/1 -> Mux1/3
  Add/1 -> Demux/1  "Position Error"
  Demux/2 -> PID_Y/1
  Mux1/1 -> Velocity Cmd/1  "Velocity Cmd"
  PID_X/1 -> Mux1/1
  PID_Y/1 -> Mux1/2
  Bus Selector1/1 -> Add/2  "<WorldPosition>"
  QuadRotorState/1 -> Bus Selector1/1
  PositionCmd/1 -> Add/1

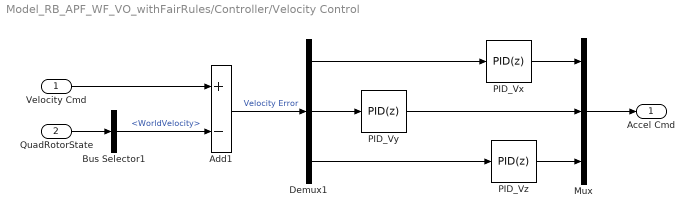
== system Model_RB_APF_WF_VO_withFairRules/Controller/Velocity Control ==
  Velocity Cmd : Inport
  QuadRotorState : Inport  Port=2
  Add1 : Sum  Inputs=+-
  Bus Selector1 : BusSelector  OutputSignals=WorldVelocity
  Demux1 : Demux  Outputs=3
  Mux : Mux  Inputs=3
  PID_Vx : slpidlib/PID Controller  Controller=PID  Form=Parallel  TimeDomain=Discrete-time  UseExternalTs=off  SampleTime=-1  IntegratorMethod=Forward Euler  FilterMethod=Forward Euler  ControllerParametersSource=internal  P=kP_vel  I=kI_vel  UseKiTs=off  D=kD_vel  UseExternalDerivativeSource=off  N=N_filter  UseFilter=on  TunerSelectOption=Transfer Function Based (PID Tuner App)  InitialConditionSource=internal  InitialConditionForIntegrator=0  InitialConditionForFilter=0  DifferentiatorICPrevScaledInput=0  ExternalReset=none  TrackingMode=off  Kt=1  LimitOutput=on  SatLimitsSource=internal  UpperSaturationLimit=1  LowerSaturationLimit=-1  LinearizeAsGain=on  AntiWindupMode=clamping  Kb=1  LimitIntegrator=off  UpperIntegratorSaturationLimit=inf  LowerIntegratorSaturationLimit=-inf  POutMin=[]  POutMax=[]  IOutMin=[]  IOutMax=[]  DOutMin=[]  DOutMax=[]  NOutMin=[]  NOutMax=[]  SumOutMin=[]  SumOutMax=[]  SaturationOutMin=[]  SaturationOutMax=[]  PParamMin=[]  PParamMax=[]  IParamMin=[]  IParamMax=[]  DParamMin=[]  DParamMax=[]  NParamMin=[]  NParamMax=[]  KbParamMin=[]  KbParamMax=[]  KtParamMin=[]  KtParamMax=[]  KbOutMin=[]  KbOutMax=[]  KtOutMin=[]  KtOutMax=[]  IntegratorOutMin=[]  IntegratorOutMax=[]  FilterOutMin=[]  FilterOutMax=[]  SumI1OutMin=SumI1OutMin  SumI1OutMax=SumI1OutMax  SumI2OutMin=[]  SumI2OutMax=[]  SumI3OutMin=[]  SumI3OutMax=[]  SumI4OutMin=[]  SumI4OutMax=[]  SumDOutMin=[]  SumDOutMax=[]  DifferentiatorOutMin=[]  DifferentiatorOutMax=[]  FilterDiffOutCoefMin=[]  FilterDiffOutCoefMax=[]  ReciprocalOutMin=[]  ReciprocalOutMax=[]  SumDenOutMin=[]  SumDenOutMax=[]  SumNumOutMin=[]  SumNumOutMax=[]  DivideOutMin=[]  DivideOutMax=[]  UdiffTsProdOutMin=[]  UdiffTsProdOutMax=[]  NTsProdOutMin=[]  NTsProdOutMax=[]  UintegralTsProdOutMin=[]  UintegralTsProdOutMax=[]  UngainTsProdOutMin=[]  UngainTsProdOutMax=[]  ClampingZeroOutDataTypeStr=Inherit: Inherit via back propagation  ClampingZeroOutMin=[]  ClampingZeroOutMax=[]  FilterDenConstantOutDataTypeStr=Inherit: Inherit via back propagation  FilterDenConstantOutMin=[]  FilterDenConstantOutMax=[]  PCopyOutDataTypeStr=Inherit: Inherit via back propagation  PCopyOutMin=[]  PCopyOutMax=[]  NCopyOutDataTypeStr=Inherit: Inherit via back propagation  NCopyOutMin=[]  NCopyOutMax=[]  IntegratorContinuousStateAttributes=''  IntegratorStateMustResolveToSignalObject=off  IntegratorRTWStateStorageClass=Auto  FilterContinuousStateAttributes=''  FilterStateMustResolveToSignalObject=off  FilterRTWStateStorageClass=Auto  ParallelPVariant=InternalParameters  IdealPVariant=Disabled  IVariant=InternalParameters  DVariant=InternalParameters  IntegratorVariant=Discrete  SatVariant=Enabled  AWVariant=DiscClampingParallel  PCopyVariant=Disabled  TRVariant=Disabled  FdbkBlocksVariant=Forward  IdealPFdbkVariant=Disabled  SatFdbkVariant=Disabled  DerivativeFilterVariant=ForwardEulerFilter  NVariant=InternalParameters  NCopyVariant=Disabled  FilterICVariant=InternalICsFilter  IntegratorICVariant=InternalICs  ExternalResetVariant=Disabled  TRSumVariant=Passthrough  SumFdbkVariant=Disabled  SumVariant=Sum_PID  TsampFilterVariant=InternalTs  TsampNgainVariant=Passthrough  TsampIntegralVariant=Disabled_SignalSpec  ExternalSaturationOutDataTypeStr=Inherit: Same as second input  DerivativeSourceVariant=ErrorSignal  PreIntVariant=InternalPreInt
      settings: AttributesFormatString=P: %<P>, I: %<I>, D:%<D>
  PID_Vy : slpidlib/PID Controller  Controller=PID  Form=Parallel  TimeDomain=Discrete-time  UseExternalTs=off  SampleTime=-1  IntegratorMethod=Forward Euler  FilterMethod=Forward Euler  ControllerParametersSource=internal  P=kP_vel  I=kI_vel  UseKiTs=off  D=kD_vel  UseExternalDerivativeSource=off  N=N_filter  UseFilter=on  TunerSelectOption=Transfer Function Based (PID Tuner App)  InitialConditionSource=internal  InitialConditionForIntegrator=0  InitialConditionForFilter=0  DifferentiatorICPrevScaledInput=0  ExternalReset=none  TrackingMode=off  Kt=1  LimitOutput=on  SatLimitsSource=internal  UpperSaturationLimit=1  LowerSaturationLimit=-1  LinearizeAsGain=on  AntiWindupMode=clamping  Kb=1  LimitIntegrator=off  UpperIntegratorSaturationLimit=inf  LowerIntegratorSaturationLimit=-inf  POutMin=[]  POutMax=[]  IOutMin=[]  IOutMax=[]  DOutMin=[]  DOutMax=[]  NOutMin=[]  NOutMax=[]  SumOutMin=[]  SumOutMax=[]  SaturationOutMin=[]  SaturationOutMax=[]  PParamMin=[]  PParamMax=[]  IParamMin=[]  IParamMax=[]  DParamMin=[]  DParamMax=[]  NParamMin=[]  NParamMax=[]  KbParamMin=[]  KbParamMax=[]  KtParamMin=[]  KtParamMax=[]  KbOutMin=[]  KbOutMax=[]  KtOutMin=[]  KtOutMax=[]  IntegratorOutMin=[]  IntegratorOutMax=[]  FilterOutMin=[]  FilterOutMax=[]  SumI1OutMin=SumI1OutMin  SumI1OutMax=SumI1OutMax  SumI2OutMin=[]  SumI2OutMax=[]  SumI3OutMin=[]  SumI3OutMax=[]  SumI4OutMin=[]  SumI4OutMax=[]  SumDOutMin=[]  SumDOutMax=[]  DifferentiatorOutMin=[]  DifferentiatorOutMax=[]  FilterDiffOutCoefMin=[]  FilterDiffOutCoefMax=[]  ReciprocalOutMin=[]  ReciprocalOutMax=[]  SumDenOutMin=[]  SumDenOutMax=[]  SumNumOutMin=[]  SumNumOutMax=[]  DivideOutMin=[]  DivideOutMax=[]  UdiffTsProdOutMin=[]  UdiffTsProdOutMax=[]  NTsProdOutMin=[]  NTsProdOutMax=[]  UintegralTsProdOutMin=[]  UintegralTsProdOutMax=[]  UngainTsProdOutMin=[]  UngainTsProdOutMax=[]  ClampingZeroOutDataTypeStr=Inherit: Inherit via back propagation  ClampingZeroOutMin=[]  ClampingZeroOutMax=[]  FilterDenConstantOutDataTypeStr=Inherit: Inherit via back propagation  FilterDenConstantOutMin=[]  FilterDenConstantOutMax=[]  PCopyOutDataTypeStr=Inherit: Inherit via back propagation  PCopyOutMin=[]  PCopyOutMax=[]  NCopyOutDataTypeStr=Inherit: Inherit via back propagation  NCopyOutMin=[]  NCopyOutMax=[]  IntegratorContinuousStateAttributes=''  IntegratorStateMustResolveToSignalObject=off  IntegratorRTWStateStorageClass=Auto  FilterContinuousStateAttributes=''  FilterStateMustResolveToSignalObject=off  FilterRTWStateStorageClass=Auto  ParallelPVariant=InternalParameters  IdealPVariant=Disabled  IVariant=InternalParameters  DVariant=InternalParameters  IntegratorVariant=Discrete  SatVariant=Enabled  AWVariant=DiscClampingParallel  PCopyVariant=Disabled  TRVariant=Disabled  FdbkBlocksVariant=Forward  IdealPFdbkVariant=Disabled  SatFdbkVariant=Disabled  DerivativeFilterVariant=ForwardEulerFilter  NVariant=InternalParameters  NCopyVariant=Disabled  FilterICVariant=InternalICsFilter  IntegratorICVariant=InternalICs  ExternalResetVariant=Disabled  TRSumVariant=Passthrough  SumFdbkVariant=Disabled  SumVariant=Sum_PID  TsampFilterVariant=InternalTs  TsampNgainVariant=Passthrough  TsampIntegralVariant=Disabled_SignalSpec  ExternalSaturationOutDataTypeStr=Inherit: Same as second input  DerivativeSourceVariant=ErrorSignal  PreIntVariant=InternalPreInt
      settings: AttributesFormatString=P: %<P>, I: %<I>, D:%<D>
  PID_Vz : slpidlib/PID Controller  Controller=PID  Form=Parallel  TimeDomain=Discrete-time  UseExternalTs=off  SampleTime=-1  IntegratorMethod=Forward Euler  FilterMethod=Forward Euler  ControllerParametersSource=internal  P=kP_vel  I=kI_vel  UseKiTs=off  D=kD_vel  UseExternalDerivativeSource=off  N=N_filter  UseFilter=on  TunerSelectOption=Transfer Function Based (PID Tuner App)  InitialConditionSource=internal  InitialConditionForIntegrator=0  InitialConditionForFilter=0  DifferentiatorICPrevScaledInput=0  ExternalReset=none  TrackingMode=off  Kt=1  LimitOutput=on  SatLimitsSource=internal  UpperSaturationLimit=4  LowerSaturationLimit=-4  LinearizeAsGain=on  AntiWindupMode=clamping  Kb=1  LimitIntegrator=off  UpperIntegratorSaturationLimit=inf  LowerIntegratorSaturationLimit=-inf  POutMin=[]  POutMax=[]  IOutMin=[]  IOutMax=[]  DOutMin=[]  DOutMax=[]  NOutMin=[]  NOutMax=[]  SumOutMin=[]  SumOutMax=[]  SaturationOutMin=[]  SaturationOutMax=[]  PParamMin=[]  PParamMax=[]  IParamMin=[]  IParamMax=[]  DParamMin=[]  DParamMax=[]  NParamMin=[]  NParamMax=[]  KbParamMin=[]  KbParamMax=[]  KtParamMin=[]  KtParamMax=[]  KbOutMin=[]  KbOutMax=[]  KtOutMin=[]  KtOutMax=[]  IntegratorOutMin=[]  IntegratorOutMax=[]  FilterOutMin=[]  FilterOutMax=[]  SumI1OutMin=SumI1OutMin  SumI1OutMax=SumI1OutMax  SumI2OutMin=[]  SumI2OutMax=[]  SumI3OutMin=[]  SumI3OutMax=[]  SumI4OutMin=[]  SumI4OutMax=[]  SumDOutMin=[]  SumDOutMax=[]  DifferentiatorOutMin=[]  DifferentiatorOutMax=[]  FilterDiffOutCoefMin=[]  FilterDiffOutCoefMax=[]  ReciprocalOutMin=[]  ReciprocalOutMax=[]  SumDenOutMin=[]  SumDenOutMax=[]  SumNumOutMin=[]  SumNumOutMax=[]  DivideOutMin=[]  DivideOutMax=[]  UdiffTsProdOutMin=[]  UdiffTsProdOutMax=[]  NTsProdOutMin=[]  NTsProdOutMax=[]  UintegralTsProdOutMin=[]  UintegralTsProdOutMax=[]  UngainTsProdOutMin=[]  UngainTsProdOutMax=[]  ClampingZeroOutDataTypeStr=Inherit: Inherit via back propagation  ClampingZeroOutMin=[]  ClampingZeroOutMax=[]  FilterDenConstantOutDataTypeStr=Inherit: Inherit via back propagation  FilterDenConstantOutMin=[]  FilterDenConstantOutMax=[]  PCopyOutDataTypeStr=Inherit: Inherit via back propagation  PCopyOutMin=[]  PCopyOutMax=[]  NCopyOutDataTypeStr=Inherit: Inherit via back propagation  NCopyOutMin=[]  NCopyOutMax=[]  IntegratorContinuousStateAttributes=''  IntegratorStateMustResolveToSignalObject=off  IntegratorRTWStateStorageClass=Auto  FilterContinuousStateAttributes=''  FilterStateMustResolveToSignalObject=off  FilterRTWStateStorageClass=Auto  ParallelPVariant=InternalParameters  IdealPVariant=Disabled  IVariant=InternalParameters  DVariant=InternalParameters  IntegratorVariant=Discrete  SatVariant=Enabled  AWVariant=DiscClampingParallel  PCopyVariant=Disabled  TRVariant=Disabled  FdbkBlocksVariant=Forward  IdealPFdbkVariant=Disabled  SatFdbkVariant=Disabled  DerivativeFilterVariant=ForwardEulerFilter  NVariant=InternalParameters  NCopyVariant=Disabled  FilterICVariant=InternalICsFilter  IntegratorICVariant=InternalICs  ExternalResetVariant=Disabled  TRSumVariant=Passthrough  SumFdbkVariant=Disabled  SumVariant=Sum_PID  TsampFilterVariant=InternalTs  TsampNgainVariant=Passthrough  TsampIntegralVariant=Disabled_SignalSpec  ExternalSaturationOutDataTypeStr=Inherit: Same as second input  DerivativeSourceVariant=ErrorSignal  PreIntVariant=InternalPreInt
      settings: AttributesFormatString=P: %<P>, I: %<I>, D:%<D>
  Accel Cmd : Outport
  wires:
  Add1/1 -> Demux1/1  "Velocity Error"
  PID_Vz/1 -> Mux/3
  Demux1/1 -> PID_Vx/1
  PID_Vy/1 -> Mux/2
  Velocity Cmd/1 -> Add1/1
  Demux1/3 -> PID_Vz/1
  Mux/1 -> Accel Cmd/1
  PID_Vx/1 -> Mux/1
  Demux1/2 -> PID_Vy/1
  Bus Selector1/1 -> Add1/2  "<WorldVelocity>"
  QuadRotorState/1 -> Bus Selector1/1

== matlab function Model_RB_APF_WF_VO_withFairRules/Path Planning Data/GoalReached_V5 ==
  settings: updateMethod=DISCRETE
  data: time input; currentWaypoint output; endSim output; pos input; waypoints input
function [currentWaypoint, endSim] = fcn(time, pos, waypoints)

waypoint_threshold = 0.25;

persistent idx;
persistent numWaypoints;
if isempty(idx)
    idx = 1;
    numWaypoints = size(waypoints, 1);
end

if norm(waypoints(idx,:).' - pos) < waypoint_threshold
    disp('Reached Waypoint');
    disp(idx);
    idx = idx + 1;
end

if idx > numWaypoints
    endSim = 1;
    currentWaypoint = waypoints(end,:).'; % can't have it empty
    disp('Sim ended at t =');
    disp(time);
    return;
end

currentWaypoint = waypoints(idx,:).';
endSim = 0;

== matlab function Model_RB_APF_WF_VO_withFairRules/Controller/MATLAB Function1 ==
  data: vel_cmd input; vel_capped output; TopSpeed input
function vel_capped = limiter(vel_cmd, TopSpeed)

mag = norm(vel_cmd);

if mag > TopSpeed
    vel_capped = TopSpeed*(vel_cmd/mag);
else
    vel_capped = vel_cmd;
end

== matlab function Model_RB_APF_WF_VO_withFairRules/WF/MATLAB Function1 ==
  data: WF_vec input; WF_VecCapped output
function WF_VecCapped = limiter(WF_vec)

maximum = 5;

mag = norm(WF_vec);

if mag > maximum
    WF_VecCapped = maximum*(WF_vec/mag);
else
    WF_VecCapped = WF_vec;
end

== matlab function Model_RB_APF_WF_VO_withFairRules/WF/WFVectors_V5 ==
  data: cloud input; virtuals input; virtualCount input; flight_mode input; pos input; radial_vec output; lateral_vec output
function [radial_vec, lateral_vec] = WF(cloud, virtuals, virtualCount, flight_mode, pos)

% Parameters
comfort_zone = 2;
lateral_scaler = 0.5;
radial_scaler = 1.5;

% Lidar cloud - find closest point
r_all    = -cloud.';
D_all    = sqrt(sum(r_all.^2, 1));
[d_min_cloud, idx_min] = min(D_all(:));
r_min_cloud = r_all(:, idx_min);

% Virtual obstacles - find closest point
if virtualCount > 0
    v_r_all = -(virtuals(1:virtualCount,:).' - pos);
    v_D_all = sqrt(sum(v_r_all.^2, 1));
    [v_d_min, v_idx_min] = min(v_D_all(:));
    v_r_min = v_r_all(:, v_idx_min);
else
    v_d_min = inf;
    v_r_min = zeros(3,1);
end

% Pick overall closest
if v_d_min < d_min_cloud
    d_min = v_d_min;
    r_min = v_r_min;
else
    d_min = d_min_cloud;
    r_min = r_min_cloud;
end

% Radial
radial_dir = r_min / d_min;             % unit vector
radial_dif = (comfort_zone - d_min);
radial_vec = radial_dir*radial_dif*radial_scaler;

% Lateral
if flight_mode == 2
    lateral_dir = [radial_dir(2); -radial_dir(1); 0];   % rotate -pi/2 about z
else
    lateral_dir = [-radial_dir(2); radial_dir(1); 0];   % rotate pi/2 about z
end

lateral_vec = lateral_dir*lateral_scaler;

== matlab function Model_RB_APF_WF_VO_withFairRules/APF/APF_Limiter1 ==
  data: del_U input; gradientCapped output
function gradientCapped = limiter(del_U)

maximum = 5;

mag = norm(del_U);

if mag > maximum
    gradientCapped = maximum*(del_U/mag);
else
    gradientCapped = del_U;
end

== matlab function Model_RB_APF_WF_VO_withFairRules/APF/APF_Limiter2 ==
  data: del_U input; gradientCapped output
function gradientCapped = limiter(del_U)

maximum = 5;

mag = norm(del_U);

if mag > maximum
    gradientCapped = maximum*(del_U/mag);
else
    gradientCapped = del_U;
end

== matlab function Model_RB_APF_WF_VO_withFairRules/APF/Attract ==
  data: q input; del_U_att output; q_goal input
function del_U_att = attractive(q, q_goal)

    % Parameters
    zeta = 0.3;           % how strongly we attract to goal
    d_star = 3;         % the point at which our attraction maxes out
                        % del_U_att max = zeta*d_star 

    % Calculate Distance
    d = norm((q_goal - q));
    
    if d <= d_star
       del_U_att = zeta*(q_goal - q);
    else 
        del_U_att = d_star*zeta*(q_goal - q)/d;
    end

    

end

== matlab function Model_RB_APF_WF_VO_withFairRules/APF/APF_Limiter ==
  data: del_U input; gradientCapped output
function gradientCapped = limiter(del_U)

maximum = 5;

mag = norm(del_U);

if mag > maximum
    gradientCapped = maximum*(del_U/mag);
else
    gradientCapped = del_U;
end

== matlab function Model_RB_APF_WF_VO_withFairRules/APF/RepulseWithVirtuals_V5 ==
  data: cloud input; virtuals input; virtualCount input; q input; del_U_rep output
function del_U_rep = repulsive(cloud, virtuals, virtualCount, q)

% Sort of 2 basic approaches. Define repulse in terms of either: ALL or CLOSEST obstacles

% Parameters
Q_star = 5;     % how far away we ignore obstacles at
eta = 0.03;    % how strongly we reppel from obstacles (how soon del_U_rep goes to infinity)
veta = 200;     % how strongly we reppel from virtual obstacles


del_U_rep = zeros(size(q));    % 3x1 vector

% Cloud Repulse
r_all = -cloud.';                          % 3xN
D_all = sqrt(sum(r_all.^2, 1));            % 1xN
in_range  = D_all <= Q_star & D_all > 0;       % 1xN logical
r_m   = r_all(:, in_range);                    % 3xM
D_m   = D_all(in_range);                       % 1xM
del_U_rep = del_U_rep + eta * sum((1./D_m - 1/Q_star) .* (1./D_m.^2) .* (r_m ./ D_m), 2);

% Virtuals Repulse
if virtualCount > 0
    v_r_all    = -(virtuals(1:virtualCount,:).' - q);
    v_D_all    = sqrt(sum(v_r_all.^2, 1));
    v_in_range = v_D_all <= Q_star & v_D_all > 0;
    v_r_m      = v_r_all(:, v_in_range);
    v_D_m      = v_D_all(v_in_range);
    del_U_rep  = del_U_rep + veta * sum((1./v_D_m - 1/Q_star) .* (1./v_D_m.^2) .* (v_r_m ./ v_D_m), 2);
end

== matlab function Model_RB_APF_WF_VO_withFairRules/Vertical Constraint/MATLAB Function ==
  data: desired_pos input; constrained_pos output; current_waypoint input
function constrained_pos = constrainZ(desired_pos, current_waypoint)

constrained_pos = [desired_pos(1); desired_pos(2); current_waypoint(3)];

== matlab function Model_RB_APF_WF_VO_withFairRules/Path Planning Data/MATLAB Function ==
  data: pts input; points output
function points = lidarToPoints(pts)

xLidar = reshape(pts(:,:,1),[],1);
yLidar = reshape(pts(:,:,2),[],1);
zLidar = reshape(pts(:,:,3),[],1);
    
points = [xLidar,yLidar,zLidar];    % Lidar points are in X,Y,Z order
